simulink model "PAC Exp3"  (R2016a)
settings: Solver=VariableStepAuto  StartTime=0.0  StopTime=10.0  RelTol=1e-3
libraries: simulink x7
settings Model: Creator=PAPUN  LastModifiedBy=PAPUN

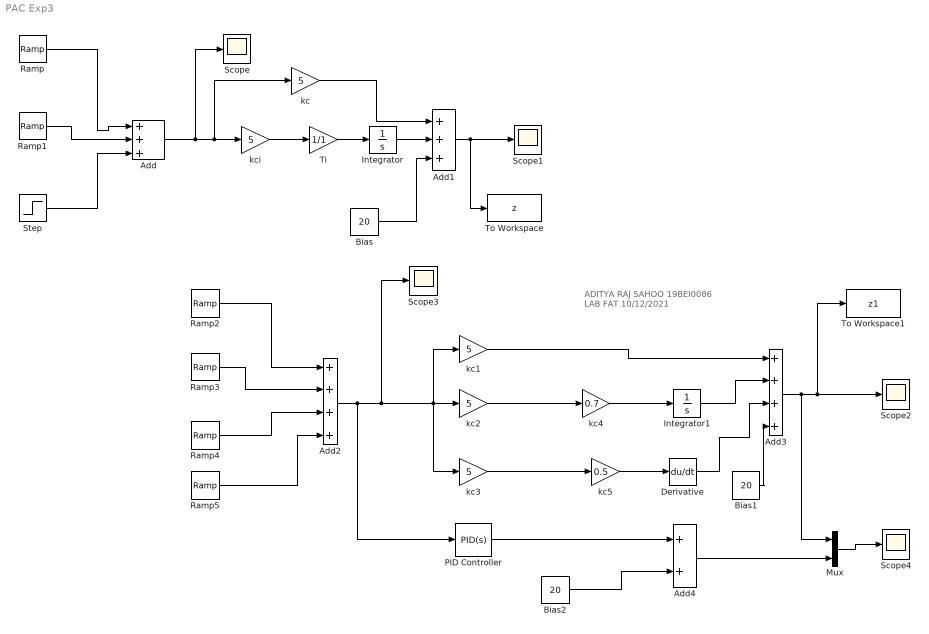
== system PAC Exp3 ==
  note: ADITYA RAJ SAHOO
      | 19BEI0086
      | LAB FAT 10/12/2021
  Add : Sum  Inputs=+++
  Add1 : Sum  Inputs=+++
  Add2 : Sum  Inputs=++++
  Add3 : Sum  Inputs=++++
  Add4 : Sum
  Bias : Constant  Value=20
  Bias1 : Constant  Value=20
  Bias2 : Constant  Value=20
  Derivative : Derivative
  Integrator : Integrator
  Integrator1 : Integrator
  Mux : Mux  Inputs=2
  PID Controller : simulink/Continuous/PID Controller  Controller=PID  TimeDomain=Continuous-time  SampleTime=-1  IntegratorMethod=Forward Euler  FilterMethod=Forward Euler  Form=Parallel  UseFilter=on  ControllerParametersSource=internal  P=5  I=3.5  D=2.5  N=500  InitialConditionSource=internal  InitialConditionForIntegrator=0  InitialConditionForFilter=0  ExternalReset=none  LimitOutput=off  UpperSaturationLimit=inf  LowerSaturationLimit=-inf  LinearizeAsGain=on  AntiWindupMode=none  Kb=1  TrackingMode=off  Kt=1  PParamMin=[]  PParamMax=[]  IParamMin=[]  IParamMax=[]  DParamMin=[]  DParamMax=[]  NParamMin=[]  NParamMax=[]  KbParamMin=[]  KbParamMax=[]  KtParamMin=[]  KtParamMax=[]  POutMin=[]  POutMax=[]  IOutMin=[]  IOutMax=[]  DOutMin=[]  DOutMax=[]  NOutMin=[]  NOutMax=[]  KbOutMin=[]  KbOutMax=[]  KtOutMin=[]  KtOutMax=[]  IntegratorOutMin=[]  IntegratorOutMax=[]  FilterOutMin=[]  FilterOutMax=[]  SumOutMin=[]  SumOutMax=[]  SumI1OutMin=[]  SumI1OutMax=[]  SumI2OutMin=[]  SumI2OutMax=[]  SumI3OutMin=[]  SumI3OutMax=[]  SumDOutMin=[]  SumDOutMax=[]  SaturationOutMin=[]  SaturationOutMax=[]  IntegratorContinuousStateAttributes=''  IntegratorStateMustResolveToSignalObject=off  IntegratorRTWStateStorageClass=Auto  FilterContinuousStateAttributes=''  FilterStateMustResolveToSignalObject=off  FilterRTWStateStorageClass=Auto  DifferentiatorICPrevScaledInput=0  DifferentiatorOutMin=[]  DifferentiatorOutMax=[]
  Ramp : simulink/Sources/Ramp  slope=1  start=0  X0=0
  Ramp1 : simulink/Sources/Ramp  slope=-1  start=1  X0=0
  Ramp2 : simulink/Sources/Ramp  slope=1  start=0  X0=0
  Ramp3 : simulink/Sources/Ramp  slope=-1  start=1  X0=0
  Ramp4 : simulink/Sources/Ramp  slope=-0.5  start=3  X0=0
  Ramp5 : simulink/Sources/Ramp  slope=0.5  start=5  X0=0
  Scope{,1..4} (5 alike) : Scope
  Step : Step  Time=3  After=-1  SampleTime=0
  Ti : Gain  Gain=1/1
  To Workspace : ToWorkspace  VariableName=z  SaveFormat=Timeseries  SampleTime=-1
  To Workspace1 : ToWorkspace  VariableName=z1  SaveFormat=Timeseries  SampleTime=-1
  kc{,1..3} (4 alike) : Gain  Gain=5
  kc4 : Gain  Gain=0.7
  kc5 : Gain  Gain=0.5
  kci : Gain  Gain=5
  wires:
  Add/1 -> Scope/1, kc/1, kci/1
  Ramp/1 -> Add/1
  Ramp1/1 -> Add/2
  Step/1 -> Add/3
  kci/1 -> Ti/1
  Bias/1 -> Add1/3
  Ti/1 -> Integrator/1
  Integrator/1 -> Add1/2
  Add1/1 -> To Workspace/1, Scope1/1
  kc/1 -> Add1/1
  Ramp2/1 -> Add2/1
  Ramp3/1 -> Add2/2
  Ramp4/1 -> Add2/3
  Ramp5/1 -> Add2/4
  Add2/1 -> PID Controller/1, Scope3/1, kc1/1, kc3/1, kc2/1
  kc1/1 -> Add3/1
  kc2/1 -> kc4/1
  kc4/1 -> Integrator1/1
  kc3/1 -> kc5/1
  Integrator1/1 -> Add3/2
  Bias1/1 -> Add3/4
  Add3/1 -> Mux/1, To Workspace1/1, Scope2/1
  kc5/1 -> Derivative/1
  Derivative/1 -> Add3/3
  PID Controller/1 -> Add4/1
  Mux/1 -> Scope4/1
  Add4/1 -> Mux/2
  Bias2/1 -> Add4/2
